simulink model "COUNTER"  (R2024a)
settings: Solver=FixedStepDiscrete  StartTime=0.0  StopTime=10.0  FixedStep=0.5  RelTol=1e-3
settings Model: Creator=prabo  LastModifiedBy=prabo

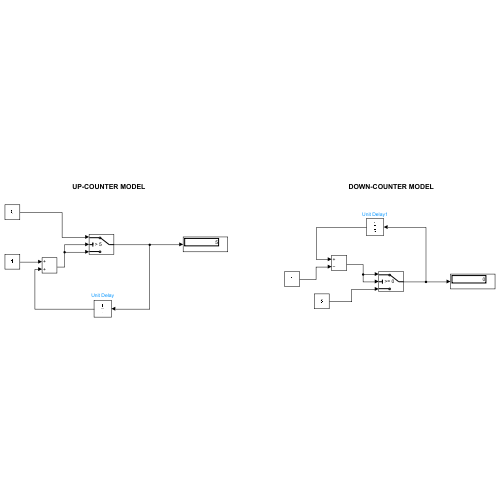
[thumbnail: Simulink's stored preview of the top-level diagram]
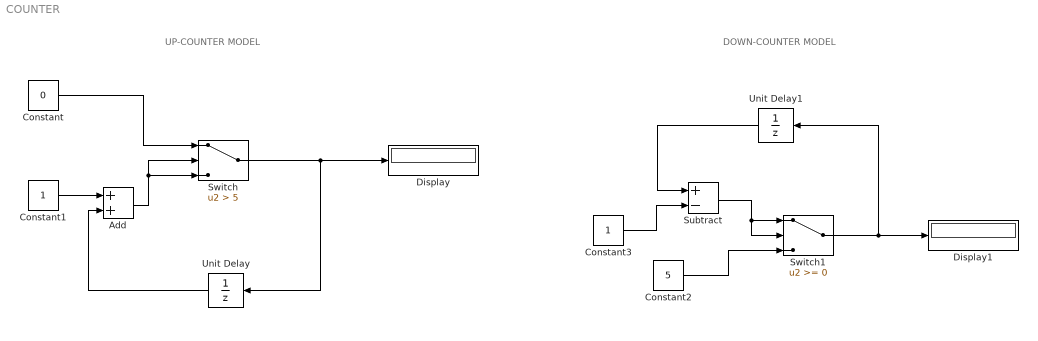
== system COUNTER ==
  note: DOWN-COUNTER MODEL
  note: UP-COUNTER MODEL
  Add : Sum
  Constant : Constant  Value=0
  Constant1 : Constant
  Constant2 : Constant  Value=5
  Constant3 : Constant
  Display : Display
  Display1 : Display
  Subtract : Sum  Inputs=+-
  Switch : Switch  Criteria=u2 > Threshold  Threshold=5  SaturateOnIntegerOverflow=off  InputSameDT=off
  Switch1 : Switch  SaturateOnIntegerOverflow=off  InputSameDT=off
  Unit Delay : UnitDelay  InitialCondition=-1  SampleTime=-1  HasFrameUpgradeWarning=on
  Unit Delay1 : UnitDelay  InitialCondition=6  SampleTime=-1  HasFrameUpgradeWarning=on
  wires:
  Constant/1 -> Switch/1
  Constant1/1 -> Add/1
  Unit Delay/1 -> Add/2
  Add/1 -> Switch/2, Switch/3
  Switch/1 -> Unit Delay/1, Display/1
  Constant2/1 -> Switch1/3
  Switch1/1 -> Unit Delay1/1, Display1/1
  Subtract/1 -> Switch1/2, Switch1/1
  Constant3/1 -> Subtract/2
  Unit Delay1/1 -> Subtract/1
